simulink model "SCIS_V3"  (R2025b)
settings: Solver=VariableStepAuto  StartTime=0.0  StopTime=318.10408521  MaxStep=3.125e-6  RelTol=1e-5  AbsTol=1e-6
libraries: fl_lib x35, nesl_utility x25, ee_lib x20
(part 2 of 2)

== matlab function SCIS_V3/MATLAB Function1 ==
  data: Time input; P output
function P = fcn(Time)
%% SCIS Frequency Sweep Generator
% Outputs period P for a logarithmically-spaced frequency sweep
% Frequencies: 40 kHz down to 1 Hz (high to low, matching EIS convention)
% Points per decade: 10
% Cycles per frequency: 20 (for FFT) + settling buffer

% Define frequency vector (log-spaced, high to low)
% 4.6 decades: 1 Hz to 40 kHz
f_start = 40000;    % Hz (start high)
f_end   = 1;        % Hz (end low)
ppd     = 10;       % points per decade
n_decades = log10(f_start/f_end);
n_points  = round(n_decades * ppd) + 1;  % ~47 points

% Generate log-spaced frequencies
f_vec = logspace(log10(f_start), log10(f_end), n_points);

% Cycles per frequency point
n_settle = 5;     % settling cycles (discard in post-processing)
n_acquire = 20;   % acquisition cycles (used for FFT)
n_total = n_settle + n_acquire;

% Calculate cumulative time boundaries
% Time for each freq = n_total / f
t_boundaries = zeros(1, n_points);
t_boundaries(1) = n_total / f_vec(1);
for k = 2:n_points
    t_boundaries(k) = t_boundaries(k-1) + n_total / f_vec(k);
end

% Determine which frequency segment we're in
P = 1/f_vec(end);  % default to lowest frequency
for k = 1:n_points
    if Time <= t_boundaries(k)
        P = 1/f_vec(k);
        break;
    end
end

end

== matlab function SCIS_V3/MATLAB Function ==
  data: Time input; P output
function P = fcn(Time)
%% SCIS Frequency Sweep Generator
% Outputs period P for a logarithmically-spaced frequency sweep
% Frequencies: 40 kHz down to 1 Hz (high to low, matching EIS convention)
% Points per decade: 10
% Cycles per frequency: 20 (for FFT) + settling buffer

% Define frequency vector (log-spaced, high to low)
% 4.6 decades: 1 Hz to 40 kHz
f_start = 40000;    % Hz (start high)
f_end   = 1;        % Hz (end low)
ppd     = 10;       % points per decade
n_decades = log10(f_start/f_end);
n_points  = round(n_decades * ppd) + 1;  % ~47 points

% Generate log-spaced frequencies
f_vec = logspace(log10(f_start), log10(f_end), n_points);

% Cycles per frequency point
n_settle = 5;     % settling cycles (discard in post-processing)
n_acquire = 20;   % acquisition cycles (used for FFT)
n_total = n_settle + n_acquire;

% Calculate cumulative time boundaries
% Time for each freq = n_total / f
t_boundaries = zeros(1, n_points);
t_boundaries(1) = n_total / f_vec(1);
for k = 2:n_points
    t_boundaries(k) = t_boundaries(k-1) + n_total / f_vec(k);
end

% Determine which frequency segment we're in
P = 1/f_vec(end);  % default to lowest frequency
for k = 1:n_points
    if Time <= t_boundaries(k)
        P = 1/f_vec(k);
        break;
    end
end

end

== matlab function SCIS_V3/MATLAB Function2 ==
  data: R1 input; R_sense output; R2 input; R3 input
function R_sense  = resistance_select(R1,R2,R3)
if R1 > 0.5
    R_sense = 0.10085;
elseif R2 > 0.5 
     R_sense = 0.01085;
elseif R3 > 0.5 
    R_sense = 0.00285;

else 
    R_sense = 1;
end

== matlab function SCIS_V3/MATLAB Function3 ==
  settings: updateMethod=DISCRETE
  data: t input; V_emf output; R_CT output; C_EDL output; V_PSU output; RB_G1 output; RB_G2 output; RB_G3 output; RB_G4 output; RB_G5 output; RB_G6 output; RS_G1 output; RS_G2 output; RS_G3 output; RS_MB output; MAIN_GATE output; is_EIS output; j_current output; op_idx output
function [V_emf,R_CT,C_EDL,V_PSU, ...
 RB_G1,RB_G2,RB_G3,RB_G4,RB_G5,RB_G6, ...
 RS_G1,RS_G2,RS_G3,RS_MB,MAIN_GATE,is_EIS,j_current,op_idx] = sweep_scheduler_V3(t)
%#codegen
%SWEEP_SCHEDULER_V3 Matched 10 kHz schedule for SCIS_Post_Processing_V6.
% Paste this ENTIRE file, including local functions, into MATLAB Function3.
% Keep the Clock input and all existing 18 output wires. No external helpers.
%
% BEFORE RUNNING: info = SCIS_Post_Processing_V6;
% Use info.stopTime for BOTH fresh simulations (start time 0):
%   Trial 1: MaxStep = 3.125e-6 s;  Trial 2: MaxStep = 1.5625e-6 s.
% MinStep stays auto. Keep solver tolerances, logging and noise identical.
% New schedule: 47 log-spaced frequencies from 10000 to 1 Hz per OP.
% Old 40 kHz logs/caches are NOT compatible with this schedule.
%
% is_EIS marks acquisition only; excitation also runs during burst settling.
% Cached arrays are constant; evaluation is otherwise stateless so rejected
% solver steps/backtracking cannot advance a persistent state machine.
% Clock-driven gate edges are not explicitly scheduled solver events.
% Code was statically checked; MATLAB/Simulink execution was unavailable.
persistent S OP cap
if isempty(S)
    [S,OP,~,cap,~]=scis_plan();
end
n=size(S,1); nf=n/5;
% Find OP using precomputed start times, including its initial settling.
op=1;
for q=2:5
    if t>=S((q-1)*nf+1,15), op=q; end
end
first=(op-1)*nf+1; last=op*nf;
V_emf=OP(op,2); R_CT=OP(op,3); C_EDL=cap;
j_current=OP(op,1); op_idx=double(op);
mask=uint32(OP(op,5)); sense=uint32(OP(op,4));
RB_G1=double(bitget(mask,1)); RB_G2=double(bitget(mask,2));
RB_G3=double(bitget(mask,3)); RB_G4=double(bitget(mask,4));
RB_G5=double(bitget(mask,5)); RB_G6=double(bitget(mask,6));
RS_G1=double(bitget(sense,1)); RS_G2=double(bitget(sense,2)); RS_G3=double(bitget(sense,3));
RS_MB=0; MAIN_GATE=1; is_EIS=0; V_PSU=S(first,7);
if t<S(first,4), return; end
if t>=S(n,6)
    V_PSU=S(n,7); % Hold last OP, no spurious sense bypass/current step.
    return;
end
% Binary search on burst start times. No logarithms/powers per solver call.
lo=first; hi=last;
while lo<hi
    mid=floor((lo+hi+1)/2);
    if t>=S(mid,4), lo=mid; else, hi=mid-1; end
end
k=lo; V_PSU=S(k,7);
phase=(t-S(k,4))*S(k,3);
MAIN_GATE=double(mod(phase,1)<0.5);
is_EIS=double(t>=S(k,5) && t<S(k,6));
end
function [S,OP,Rohm,C,ESR] = scis_plan()
% EDIT THIS IDENTICAL SECTION IN BOTH FILES when changing the circuit/sweep.
% All resistance values below are in OHMS. Physical blocks must match them.
Rbank = [50 30 15 10 4 2]*1e-3; % RB_G1 ... RB_G6, physical resistor values
Rsense=[100 10 2]*1e-3;        % RS_G1 ... RS_G3, keep existing sense calibration
Ron=0.85e-3; Goff=1e-6; Gdiode=1e-5;
Rohm=0.0212; C=0.4573; ESR=1e-6;
% Columns: j [A/cm2], E [V], Rct [Ohm], sense mask, perturbation mask.
% Branch weights: G1=1, G2=2, G3=4, G4=8, G5=16, G6=32.
% Fixed combinations give about 7% maximum p-p across the configured sweep.
OP = [
    0.05, 1.4270, 0.09887, 1, (1 + 2 + 8);       % G1 + G2 + G4
    0.10, 1.4504, 0.03597, 1, (2 + 8);           % G2 + G4
    0.50, 1.4814, 0.01030, 2, (2 + 4 + 8 + 16);  % G2 + G3 + G4 + G5
    1.00, 1.4970, 0.00607, 2, (1 + 32);          % G1 + G6
    4.00, 1.5250, 0.00287, 4, (2 + 4 + 32)       % G2 + G3 + G6
];
area=5; fmax=10000; fmin=1; nf=47;
acquireCycles=8; minSettleCycles=3; relaxConstants=10; opSettle=0.5;
sourceFilterTau=0.001; % Existing voltage-source input filters
% 47 logarithmic frequencies, descending from 10 kHz to 1 Hz.
% Keep this complete plan and its helpers identical in both files.
f=logspace(log10(fmax),log10(fmin),nf);
% Numeric table: no growing structure arrays.
% 1 OP, 2 freq index, 3 Hz, 4 burst start, 5 acquisition start, 6 end,
% 7 PSU V, 8 sense equivalent, 9 low bank R, 10 high bank R,
% 11 predicted p-p fraction, 12 target I, 13 acquire cycles,
% 14 settle cycles, 15 OP start, 16 fastest loaded RC time constant.
S=zeros(5*nf,16); now=0;
for op=1:5
    rs=bankR(OP(op,4),false,Rsense,Ron,Goff,Gdiode);
    rl=bankR(OP(op,5),true,Rbank,Ron,Goff,Gdiode);
    rh=bankR(OP(op,5),false,Rbank,Ron,Goff,Gdiode);
    opStart=now; now=now+opSettle;
    for k=1:nf
        [meanI,pp,tau]=periodic(f(k),rl,rh,OP(op,3),C,Rohm,rs,ESR);
        ns=max(minSettleCycles,ceil(f(k)*relaxConstants*max([tau sourceFilterTau])));
        target=area*OP(op,1); vs=OP(op,2)+target/meanI;
        a=now+ns/f(k); b=now+(ns+acquireCycles)/f(k);
        S((op-1)*nf+k,:)=[op k f(k) now a b vs rs rl rh pp target acquireCycles ns opStart min(tau)];
        now=b;
    end
end
end
function r=bankR(code,bypass,R,Ron,Goff,Gdiode)
g=0;
for k=1:numel(R)
    if bitget(uint32(code),k), sw=1/(1/Ron+Gdiode);
    else, sw=1/(Goff+Gdiode); end
    g=g+1/(R(k)+sw);
end
if bypass, g=g+1/Ron+Gdiode; else, g=g+Goff+Gdiode; end
r=1/g;
end
function [meanI,pp,tau]=periodic(f,rl,rh,Rct,C,Rohm,rs,ESR)
% Exact periodic solution for unit supply overdrive U=Vpsu-E=1 V.
% Valid for this voltage-fed linear EEC with reverse-biased MOSFET body diodes.
re=Rohm+rs+[rl rh]; D=re*Rct+(re+Rct)*ESR;
tau=C*D./(re+Rct); xi=Rct./(re+Rct);
ci=(Rct+ESR)./D; cx=Rct./D; h=.5/f;
a=exp(-h./tau); b=-expm1(-h./tau);
x0=(xi(2)*b(2)+a(2)*xi(1)*b(1))/(-expm1(-h*sum(1./tau)));
x1=xi(1)+(x0-xi(1))*a(1);
xint=xi*h+([x0 x1]-xi).*tau.*b;
meanI=sum(ci*h-cx.*xint)/(2*h);
v=[ci(1)-cx(1)*x0 ci(1)-cx(1)*x1 ci(2)-cx(2)*x1 ci(2)-cx(2)*x0];
pp=(max(v)-min(v))/meanI;
end

== matlab function SCIS_V3/MATLAB Function5 ==
  data: t input; V_emf output; R_CT output; C_EDL output; V_PSU output; RB_G1 output; RB_G2 output; RB_G3 output; RB_G4 output; RB_G5 output; RS_G1 output; RS_G2 output; RS_G3 output; RS_MB output; MAIN_GATE output; is_EIS output; j_current output; op_idx output
function [V_emf, R_CT, C_EDL, V_PSU, ...
         RB_G1, RB_G2, RB_G3, RB_G4, RB_G5, ...
         RS_G1, RS_G2, RS_G3, RS_MB, ...
         MAIN_GATE, is_EIS, j_current, op_idx] = sweep_scheduler(t)
% ========================================================================
% sweep_scheduler — SCIS Sweep Controller + Frequency Generator
% ========================================================================
% Standalone MATLAB Function block. Combines operating point scheduling,
% logarithmic frequency sweep generation, perturbation bank control,
% auto-ranging sense bank control, sense bypass management, and direct
% main bypass MOSFET gate signal generation.
%
% V3 UPDATE: MAIN_GATE replaces MAIN_BYPASS_P
%   The Variable Pulse Generator block has been eliminated. This function
%   now outputs the main bypass MOSFET gate signal directly (0 or 1)
%   using mod() to generate the square wave during EIS.
%
%   Simulink changes required:
%     1. Delete the Variable Pulse Generator block and the > 0.5 comparator
%     2. Rename the output port from MB_P to MAIN_GATE (or just rewire)
%     3. Wire MAIN_GATE directly to the MAIN BYPASS MOSFET gate input
%
% All parameters hardcoded from NREL Round Robin data (Table S1.6,
% 5 cm^2 cell, corrected j=0.01 first point).
%
% Input:  t  — simulation time (s) from Clock block
%
% Outputs:
%   V_emf          — back-EMF for Controlled Voltage Source (V)
%   R_CT           — charge-transfer resistance (Ohms)
%   C_EDL          — double-layer capacitance (F) [constant]
%   V_PSU          — PSU supply voltage (V)
%
%   RB_G1..RB_G5   — perturbation bank gate signals (0 or 1)
%                     G1 = 8 mOhm       (j = 0.05)
%                     G2 = 3 mOhm       (j = 0.10 - 0.15)
%                     G3 = 2 mOhm       (j = 0.20 - 0.30)
%                     G4 = 1.5 mOhm     (j = 0.50 - 0.80, 2x3 par)
%                     G5 = 1 mOhm       (j = 1.00 - 4.00)
%                     Settling: all ON (bypass). EIS: exclusive selection.
%
%   RS_G1..RS_G3   — sense bank gate signals (0 or 1, exclusive)
%                     G1 = 100 mOhm     (LOW,  I <= 1 A)
%                     G2 = 10  mOhm     (MID,  1 - 5 A)
%                     G3 = 2   mOhm     (HIGH, 5 - 20 A)
%                     Selected at OP start, held through settle + EIS.
%                     All OFF during post-sweep idle (RS_MB handles path).
%
%   RS_MB          — sense bank main bypass MOSFET (0 or 1)
%                     0 = OFF (sense branch active, settle + EIS)
%                     1 = ON  (bypass, lowest R path, non-EIS / idle)
%
%   MAIN_GATE      — main bypass MOSFET gate signal (0 or 1)
%                     Settling / idle: 1 (MOSFET ON, bypass active)
%                     EIS: 50% duty cycle square wave at f_current
%                       1 = MOSFET ON  (bypass, low R path)
%                       0 = MOSFET OFF (current through selected shunt)
%
%   is_EIS         — 1 = capture data, 0 = settling or idle
%   j_current      — current density (A/cm^2) for logging (0 = idle)
%   op_idx         — operating point index (1-5, or 0 = idle)
%
% State Machine:
%   +--------------+----------+--------+--------+-----------+-----------+
%   | State        | RB_G1-5  | RS_Gx  | RS_MB  | MAIN_GATE | is_EIS    |
%   +--------------+----------+--------+--------+-----------+-----------+
%   | SETTLING     | all ON   | 1 sel. | 0 OFF  | 1 (ON)    | 0         |
%   | EIS          | 1 sel.   | 1 sel. | 0 OFF  | toggling  | 1         |
%   | POST-SWEEP   | all ON   | all OFF| 1 ON   | 1 (ON)    | 0         |
%   +--------------+----------+--------+--------+-----------+-----------+
%
% Timing:
%   t_settle = 30 s,  t_EIS = 120 s,  t_per_OP = 150 s
%   5 OPs x 150 s = 750 s total sweep duration
%   t >= 750 s: post-sweep idle (all bypass)
%
% Frequency sweep: 40 kHz -> 1 Hz, 10 pts/decade, 47 frequencies
%   Each frequency: 5 settling + 20 acquisition = 25 cycles
%   Sweep resets at the start of each OP's EIS phase
%
% Source: NREL PEMWE Round Robin (Table S1.6, LL1.6 Figure S2.8d)
%         Cell: 5 cm^2, 80 deg C, Nafion N117, IrOx/Pt-C
%         R_mem  = 21.13 mOhm  (HFR avg 105.7 mOhm.cm^2 / 5 cm^2)
%         C_EDL  = 0.4573 F    (CV after conditioning, LL1.6)
%         R_DS(on) = 0.85 mOhm (BSC010N04LS at VGS = 10 V)
%
% Author: H. Finn, University of Tasmania, June 2026
% ========================================================================
%#codegen

    %% =====================================================================
    %  TIMING CONSTANTS
    %  =====================================================================
    t_settle = 30;      % seconds settling per OP
    t_EIS    = 125;     % seconds EIS characterisation per OP
    t_per_OP = 155;     % = t_settle + t_EIS
    n_OPs    = 5;       % number of operating points in sweep
    t_sweep  = n_OPs * t_per_OP;  % 750 s total sweep duration

    %% =====================================================================
    %  FREQUENCY SWEEP DEFINITION
    %  =====================================================================
    f_start       = 40000;  % Hz (start high, EIS convention)
    f_end         = 1;      % Hz (end low)
    ppd           = 10;     % points per decade
    n_decades     = log10(f_start / f_end);           % 4.602
    n_points      = round(n_decades * ppd) + 1;       % 47 frequencies
    n_settle_cyc  = 5;      % settling cycles per freq (discarded)
    n_acquire_cyc = 20;     % acquisition cycles per freq (for DFT)
    n_total_cyc   = n_settle_cyc + n_acquire_cyc;     % 25 total

    %% =====================================================================
    %  CONSTANT PARAMETER
    %  =====================================================================
    C_EDL = 0.4573;   % F (from CV measurement, LL1.6)

    %% =====================================================================
    %  POST-SWEEP IDLE CHECK
    %  =====================================================================
    if t >= t_sweep
        V_emf     = 1.5250;
        R_CT      = 0.00287;
        V_PSU     = 2.0690;
        j_current = 0;
        op_idx    = 0;
        is_EIS    = 0;

        RB_G1 = 1;  RB_G2 = 1;  RB_G3 = 1;  RB_G4 = 1;  RB_G5 = 1;

        RS_G1 = 0;  RS_G2 = 0;  RS_G3 = 0;
        RS_MB = 1;

        MAIN_GATE = 1;   % held ON (bypass)

        return;
    end

    %% =====================================================================
    %  OPERATING POINT SELECTION (within sweep)
    %  =====================================================================
    op_idx  = min(floor(t / t_per_OP) + 1, n_OPs);
    t_in_OP = t - (op_idx - 1) * t_per_OP;
    is_EIS  = double(t_in_OP >= t_settle);

    %% =====================================================================
    %  SENSE BYPASS: OFF for entire OP (settle + EIS)
    %  =====================================================================
    RS_MB = 0;

    %% =====================================================================
    %  EEC + BANK + SENSE PARAMETERS PER OPERATING POINT
    %  =====================================================================
    if op_idx <= 1
        % OP 1: j = 0.05 A/cm²,  I_target = 0.25 A
        % V_cell = 1.457 V (NREL),  Z_DC = 120.0 mΩ
        % Bank: RB_G1 (8 mΩ), Sense: RS_G1 (100 mΩ)
        j_current  = 0.05;
        V_emf      = 1.4270;       % = V_cell - I × Z_DC
        R_CT       = 0.09887;      % = Z_DC - R_mem
        V_PSU      = 1.4823;       % = V_emf + I × R_total_settle
        rb_select  = 1;
        rs_select  = 1;

    elseif op_idx == 2
        % OP 2: j = 0.10 A/cm²,  I_target = 0.50 A
        % V_cell = 1.479 V (NREL),  Z_DC = 57.1 mΩ
        j_current  = 0.10;
        V_emf      = 1.4504;
        R_CT       = 0.03597;
        V_PSU      = 1.5295;       % = V_emf + I × R_total_settle
        rb_select  = 2;
        rs_select  = 1;

    elseif op_idx == 3
        % OP 3: j = 0.50 A/cm²,  I_target = 2.50 A
        % V_cell = 1.560 V (NREL),  Z_DC = 31.4 mΩ
        j_current  = 0.50;
        V_emf      = 1.4814;
        R_CT       = 0.01030;
        V_PSU      = 1.5880;       % = V_emf + I × R_total_settle
        rb_select  = 4;
        rs_select  = 2;

    elseif op_idx == 4
        % OP 4: j = 1.00 A/cm²,  I_target = 5.00 A
        % V_cell = 1.633 V (NREL),  Z_DC = 27.2 mΩ
        j_current  = 1.00;
        V_emf      = 1.4970;
        R_CT       = 0.00607;
        V_PSU      = 1.6890;       % = V_emf + I × R_total_settle
        rb_select  = 5;
        rs_select  = 2;

    else
        % OP 5: j = 4.00 A/cm²,  I_target = 20.00 A
        % V_cell = 2.005 V (NREL),  Z_DC = 24.0 mΩ
        j_current  = 4.00;
        V_emf      = 1.5250;
        R_CT       = 0.00287;
        V_PSU      = 2.0690;       % = V_emf + I × R_total_settle
        rb_select  = 5;
        rs_select  = 3;
    end

    %% =====================================================================
    %  GATE SIGNALS: PERTURBATION BANK
    %  =====================================================================
    if is_EIS == 0
        RB_G1 = 1;  RB_G2 = 1;  RB_G3 = 1;  RB_G4 = 1;  RB_G5 = 1;
    else
        RB_G1 = double(rb_select == 1);
        RB_G2 = double(rb_select == 2);
        RB_G3 = double(rb_select == 3);
        RB_G4 = double(rb_select == 4);
        RB_G5 = double(rb_select == 5);
    end

    %% =====================================================================
    %  GATE SIGNALS: SENSE BANK (held through settle + EIS)
    %  =====================================================================
    RS_G1 = double(rs_select == 1);
    RS_G2 = double(rs_select == 2);
    RS_G3 = double(rs_select == 3);

    %% =====================================================================
    %  MAIN BYPASS GATE: DIRECT SQUARE-WAVE GENERATION
    %  =====================================================================
    %  Replaces the Variable Pulse Generator block entirely.
    %  Gate signal is computed directly using mod() — no persistent
    %  variables, no external blocks, no period-trap risk.
    %
    %  During settling: gate = 1 (MOSFET ON, bypass, DC steady state)
    %    - No switching events generated
    %    - Solver steps freely through 30 s with no forced refinement
    %    - This is why runtime is fast: zero transitions during settling
    %
    %  During EIS: gate toggles at f_current with 50% duty cycle
    %    - mod(t_local, period) produces a sawtooth 0..period
    %    - Comparison to 0.5*period produces the square wave
    %    - Phase discontinuities at frequency transitions are absorbed
    %      by the 5 settling cycles (discarded in post-processing DFT)
    %
    %  Gate convention (matches original pulse generator behaviour):
    %    1 = MOSFET ON  = bypass active   = low R path
    %    0 = MOSFET OFF = current through selected shunt branch

    if is_EIS == 0
        % SETTLING / between OPs: gate held ON, no switching events
        MAIN_GATE = 1;
    else
        % EIS ACTIVE: log sweep 40 kHz -> 1 Hz, resets each OP
        t_eis_local = t_in_OP - t_settle;

        % --- Determine current frequency from sweep schedule ---
        t_cumulative = 0;
        f_current = f_end;   % default: hold at 1 Hz after sweep ends

        for k = 1:n_points
            fk = f_start * 10^(-n_decades * (k - 1) / (n_points - 1));
            dt_k = n_total_cyc / fk;
            t_cumulative = t_cumulative + dt_k;

            if t_eis_local <= t_cumulative
                f_current = fk;
                break;
            end
        end

        % --- Generate gate signal: 50% duty cycle square wave ---
        period = 1 / f_current;
        MAIN_GATE = double(mod(t_eis_local, period) < 0.5 * period);
    end

end
